simulink model "Average_switch_model"  (R2018a)
settings: Solver=VariableStepAuto  StartTime=0.0  StopTime=0.1  RelTol=1e-3
libraries: powerlib x11
settings Model: Creator=Asus  LastModifiedBy=Asus

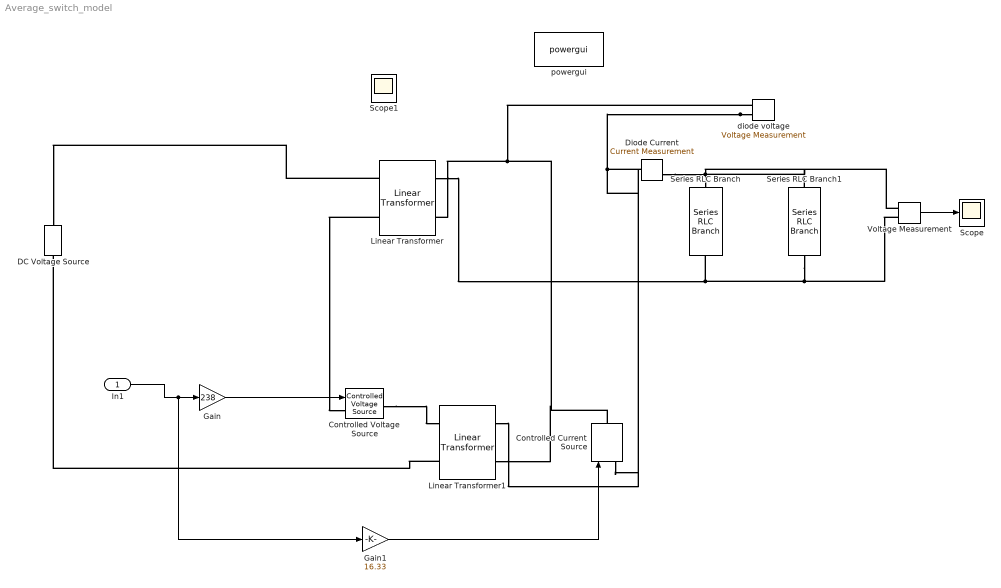
== system Average_switch_model ==
  In1 : Inport
  Controlled Current Source : powerlib/Electrical Sources/Controlled Current Source  Initialize=on  Source_Type=AC  Amplitude=0  Phase=0  Frequency=0  Measurements=None
  Controlled Voltage Source : powerlib/Electrical Sources/Controlled Voltage Source  Initialize=on  Source_Type=AC  Amplitude=0  Phase=0  Frequency=0  Measurements=None
  DC Voltage Source : powerlib/Electrical Sources/DC Voltage Source  Amplitude=36  Measurements=None
  Diode Current : powerlib/Measurements/Current Measurement  PhasorSimulation=off  OutputType=Complex  PSBequivalent=0
  Gain : Gain  Gain=238
  Gain1 : Gain  Gain=16.33
  Linear Transformer : powerlib/Elements/Linear Transformer  UNITS=SI  NominalPower=[ 100 40000 ]  winding1=[15 0 0]  winding2=[10 0 0]  ThreeWindings=off  winding3=[3.15e+05 0.7938 0.084223]  RmLm=[1.0805e+06 77e-6]  Measurements=Magnetization current  DataType=on
  Linear Transformer1 : powerlib/Elements/Linear Transformer  UNITS=SI  NominalPower=[ 100 40000 ]  winding1=[0.572 0 0]  winding2=[0.2853 0 0]  ThreeWindings=off  winding3=[3.15e+05 0.7938 0.084223]  RmLm=[1.0805e+06 inf]  Measurements=All voltages and currents  DataType=on
  Scope : Scope
  Scope1 : Scope
  Series RLC Branch : powerlib/Elements/Series RLC Branch  LConnTagsString=__new0  RConnTagsString=__new0  BranchType=RC  Resistance=0.015  Inductance=1e-3  SetiL0=off  InitialCurrent=0  Capacitance=330e-6  Setx0=off  InitialVoltage=0  Measurements=None
  Series RLC Branch1 : powerlib/Elements/Series RLC Branch  LConnTagsString=__new0  RConnTagsString=__new0  BranchType=R  Resistance=15/4  Inductance=1e-3  SetiL0=off  InitialCurrent=0  Capacitance=1e-6  Setx0=off  InitialVoltage=0  Measurements=None
  Voltage Measurement : powerlib/Measurements/Voltage Measurement  PhasorSimulation=off  OutputType=Complex  PSBequivalent=0
  diode voltage : powerlib/Measurements/Voltage Measurement  PhasorSimulation=off  OutputType=Complex  PSBequivalent=0
  powergui : powerlib/powergui  Priority=1  SimulationMode=Continuous  SampleTime=50e-6  frequency=60  Iterations=50  frequencyindice=0  Pbase=100e6  ErrMax=1e-4  UnitsV=kV  UnitsW=MW  buscounter=0  FunctionMessages=off  echomessages=off  EnableUseOfTLC=off  CurrentSourceSwitches=off  DisableSnubberDevices=off  DisableRonSwitches=off  DisableVfSwitches=off  DisplayEquations=off  SolverType=Tustin/Backward Euler (TBE)  Interpol=off  ExternalGateDelay=off  methode=off  Ts=100  x0status=blocks  SPID=on  SwTol=0  HookPort=off  RestoreLinks=warning  ResistiveCurrentMeasurement=off  Frange=[0:2:500]  Ylog=off  Xlog=on  ShowGrid=off  save=off  variable=ZData  structure=0  ZoomFFT=off  StartTime=0.0  cycles=1  DisplayStyle=1  fundamental=60  FreqAxis=off  MaxFrequency=1000  frequencyindicesteady=1  RmsSteady=1  display=off
  wires:
  Voltage Measurement/1 -> Scope/1
  Gain/1 -> Controlled Voltage Source/1
  In1/1 -> Gain1/1, Gain/1
  Gain1/1 -> Controlled Current Source/1
  connections:
  Linear Transformer/LConn1 -- DC Voltage Source/RConn1
  Linear Transformer/LConn2 -- Controlled Voltage Source/LConn1
  Series RLC Branch1/RConn1 -- Voltage Measurement/LConn2 -- Series RLC Branch/RConn1 -- Linear Transformer/RConn1
  Voltage Measurement/LConn1 -- Series RLC Branch1/LConn1 -- Diode Current/RConn1 -- Series RLC Branch/LConn1
  Linear Transformer1/LConn2 -- DC Voltage Source/LConn1
  diode voltage/LConn1 -- Linear Transformer1/RConn2 -- Controlled Current Source/RConn1 -- Linear Transformer/RConn2
  diode voltage/LConn2 -- Controlled Current Source/LConn1 -- Linear Transformer1/RConn1 -- Diode Current/LConn1
  Controlled Voltage Source/RConn1 -- Linear Transformer1/LConn1
